simulink model "Qa"  (R2021a)
settings: Solver=FixedStepAuto  StartTime=0.0  StopTime=10.0  FixedStep=0.01  RelTol=1e-3
libraries: simulink x2
settings Model: Creator=Personal Account  LastModifiedBy=Personal Account

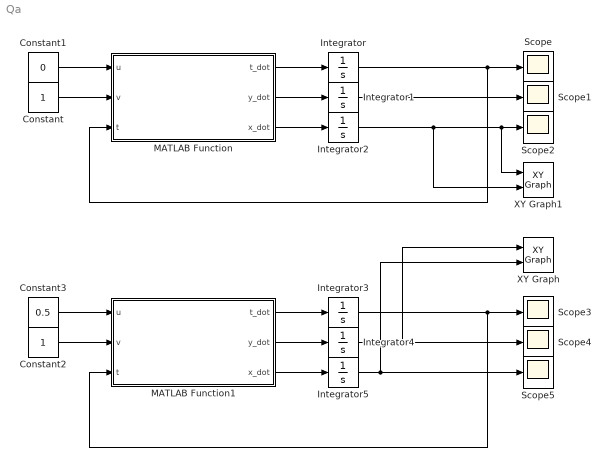
== system Qa ==
  Constant : Constant
  Constant1 : Constant  Value=0
  Constant2 : Constant
  Constant3 : Constant  Value=0.5
  Integrator{,1..5} (6 alike) : Integrator
  MATLAB Function : MATLAB Function  TreatAsAtomicUnit=on
  MATLAB Function1 : MATLAB Function  TreatAsAtomicUnit=on
  Scope{,1..5} (6 alike) : Scope
  XY Graph : simulink/Sinks/XY Graph  xmin=-10  xmax=10  ymin=-10  ymax=10  st=-1
  XY Graph1 : simulink/Sinks/XY Graph  xmin=-10  xmax=10  ymin=-10  ymax=10  st=-1
  wires:
  MATLAB Function/3(x_dot) -> Integrator2/1
  MATLAB Function/2(y_dot) -> Integrator1/1
  MATLAB Function/1(t_dot) -> Integrator/1
  Integrator/1 -> Scope/1, MATLAB Function/3(t)
  Integrator1/1 -> Scope1/1
  Integrator2/1 -> XY Graph1/2, XY Graph1/1, Scope2/1
  Constant/1 -> MATLAB Function/2(v)
  Constant1/1 -> MATLAB Function/1(u)
  Integrator3/1 -> Scope3/1, MATLAB Function1/3(t)
  MATLAB Function1/2(y_dot) -> Integrator4/1
  Integrator4/1 -> XY Graph/1, Scope4/1
  MATLAB Function1/1(t_dot) -> Integrator3/1
  Constant2/1 -> MATLAB Function1/2(v)
  Integrator5/1 -> XY Graph/2, Scope5/1
  Constant3/1 -> MATLAB Function1/1(u)
  MATLAB Function1/3(x_dot) -> Integrator5/1

== matlab function Qa/MATLAB Function1 ==
  data: u input; t_dot output; v input; t input; y_dot output; x_dot output
function [t_dot, y_dot, x_dot] = Mathematical_Model(u,v,t)
    G = [cos(t) 0;
         sin(t) 0;
         0 1];
    y = G * [v;u];
    t_dot = y(3);
    y_dot = y(2);
    x_dot = y(1);

== matlab function Qa/MATLAB Function ==
  data: u input; t_dot output; v input; t input; y_dot output; x_dot output
function [t_dot, y_dot, x_dot] = Mathematical_Model(u,v,t)
    G = [cos(t) 0;
         sin(t) 0;
         0 1];
    y = G * [v;u];
    t_dot = y(3);
    y_dot = y(2);
    x_dot = y(1);
